simulink model "primary_system"  (R2020b)
settings: Solver=VariableStepAuto  StartTime=0.0  StopTime=10.0  RelTol=1e-3
settings Model: Creator=lenovo  LastModifiedBy=lenovo

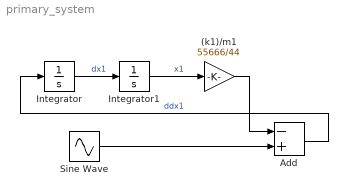
== system primary_system ==
  (k1)/m1 : Gain  Gain=55666/44
  Add : Sum  Inputs=-+
  Integrator : Integrator
  Integrator1 : Integrator
  Sine Wave : Sin  Amplitude=(0.244*0.05*(20.3)^2)/44  Frequency=20.3  SampleTime=0
  wires:
  (k1)/m1/1 -> Add/1
  Integrator1/1 -> (k1)/m1/1  "x1"
  Add/1 -> Integrator/1  "ddx1"
  Sine Wave/1 -> Add/2
  Integrator/1 -> Integrator1/1  "dx1"
